simulink model "Exp_200_TestingSystemIdent"  (R2016a)
settings: Solver=ode45  StartTime=0.0  StopTime=700  RelTol=1e-3
StartFcn:
  | clear all
settings Model: Creator=johnh  LastModifiedBy=tiago
settings DataIOCC: SaveFormat=StructureWithTime
settings HardwareCC: ProdWordSize=32  ProdHWDeviceType=Specified
settings ConfigComp: CovModelRefEnable=Off

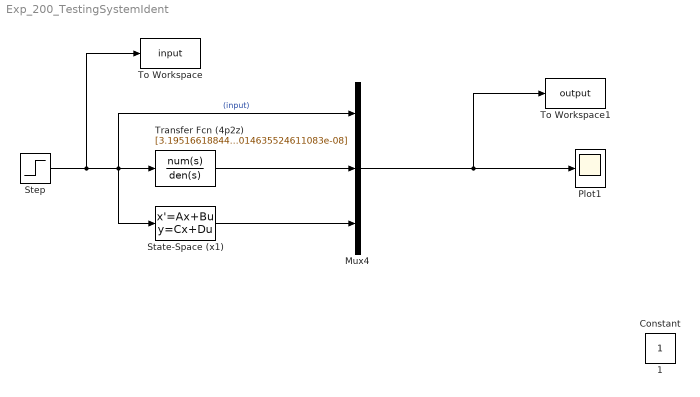
== system Exp_200_TestingSystemIdent ==
  Mux4 : Mux  Inputs=3
  Plot1 : Scope
  State-Space (x1) : StateSpace  A=-0.005070611210911  B=1.068970183519867e-05  C=3.695395325035177e+02  D=0  X0=0.004775767159700
  Step : Step  Time=50  After=70  SampleTime=0
  To Workspace : ToWorkspace  VariableName=input  SaveFormat=Timeseries  SampleTime=-1
  To Workspace1 : ToWorkspace  VariableName=output  SaveFormat=Timeseries  SampleTime=-1
  Transfer Fcn (4p2z) : TransferFcn  Numerator=[3.195166188443881e-04,-7.093012858467532e-08,6.765608163907508e-08]  Denominator=[1,0.061707735245560,6.381421465415211e-04,1.302629951453399e-05,9.014635524611083e-08]
  1 : Constant  IOType=siggen
  Constant : Constant  IOType=siggen
  wires:
  Step/1 -> To Workspace/1, State-Space (x1)/1, Mux4/1, Transfer Fcn (4p2z)/1  "(input)"
  State-Space (x1)/1 -> Mux4/3
  Transfer Fcn (4p2z)/1 -> Mux4/2
  Mux4/1 -> To Workspace1/1, Plot1/1
